simulink model "Central_locking"  (R2017b)
settings: Solver=VariableStepAuto  StartTime=0.0  StopTime=10.0  RelTol=1e-3
undefined symbols (not defined in the file): sigbuilder_block
settings Model: Creator=ECoDe_user18  LastModifiedBy=ECoDe_user11
settings ConfigComp: CovEnable=on  RecordCoverage=on  CovMetricSettings=dcmwe  CovModelRefEnable=on  CovExternalEMLEnable=off  CovSFcnEnable=off

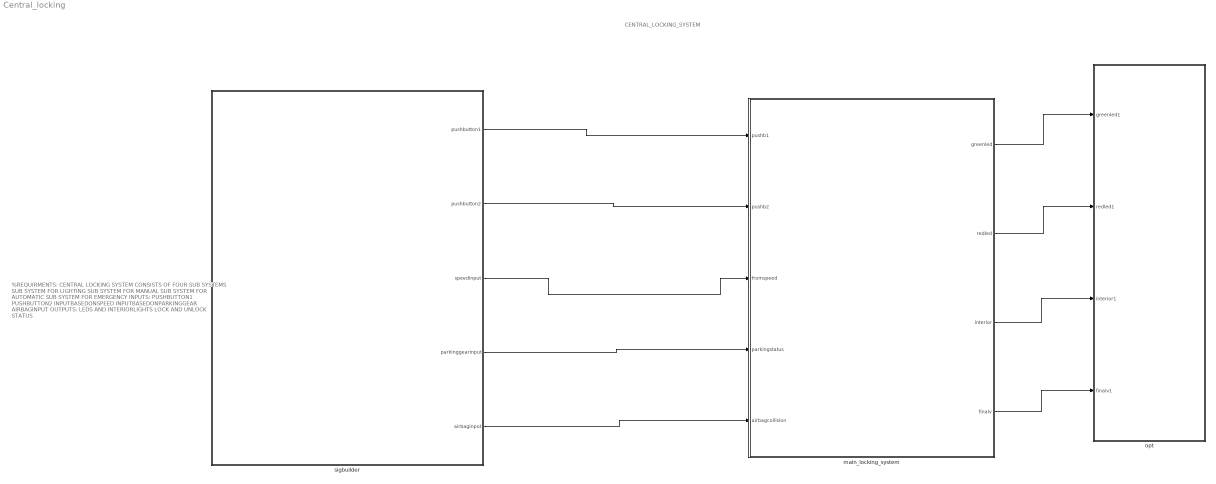
== system Central_locking ==
  note: %REQUIRMENTS:
      | CENTRAL LOCKING SYSTEM
      | CONSISTS OF FOUR SUB SYSTEMS
      | SUB SYSTEM FOR LIGHTING
      | SUB SYSTEM FOR MANUAL
      | SUB SYSTEM FOR AUTOMATIC
      | SUB SYSTEM FOR EMERGENCY
      | INPUTS:
      | PUSHBUTTON1
      | PUSHBUTTON2
      | INPUTBASEDONSPEED
      | INPUTBASEDONPARKINGGEAR
      | AIRBAGINPUT
      | OUTPUTS:
      | LEDS AND INTERIORLIGHTS
      | LOCK AND UNLOCK STATUS
  note: CENTRAL_LOCKING_SYSTEM
  main_locking_system : Subsystem
  opt : Subsystem
  sigbuilder : Subsystem
  wires:
  sigbuilder/1(pushbutton1) -> main_locking_system/1(pushb1)
  sigbuilder/2(pushbutton2) -> main_locking_system/2(pushb2)
  sigbuilder/3(speedinput) -> main_locking_system/3(fromspeed)
  sigbuilder/4(parkinggearinput) -> main_locking_system/4(parkingstatus)
  sigbuilder/5(airbaginput) -> main_locking_system/5(airbagcollision)
  main_locking_system/1(greenled) -> opt/1(greenled1)
  main_locking_system/2(redled) -> opt/2(redled1)
  main_locking_system/3(interior) -> opt/3(interior1)
  main_locking_system/4(finalv) -> opt/4(finalv1)

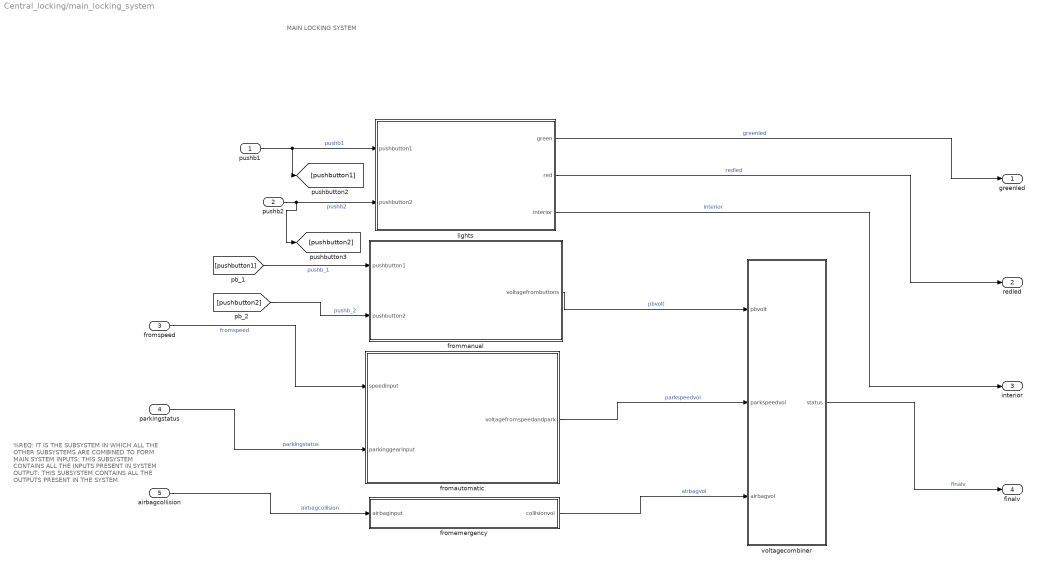
== system Central_locking/main_locking_system ==
  note: %REQ:
      | IT IS THE SUBSYSTEM IN
      | WHICH ALL THE OTHER SUBSYSTEMS
      | ARE COMBINED TO FORM MAIN SYSTEM
      | INPUTS:
      | THIS SUBSYSTEM CONTAINS ALL THE
      | INPUTS PRESENT IN SYSTEM
      | OUTPUT:
      | THIS SUBSYSTEM CONTAINS ALL THE
      | OUTPUTS PRESENT IN  THE SYSTEM.
  note: MAIN LOCKING SYSTEM
  pushb1 : Inport
  pushb2 : Inport  Port=2
  fromspeed : Inport  Port=3
  parkingstatus : Inport  Port=4
  airbagcollision : Inport  Port=5
  fromautomatic : Subsystem
  fromemergency : Subsystem
  frommanual : Subsystem
  lights : Subsystem
  voltagecombiner : Subsystem
  greenled : Outport
  redled : Outport  Port=2
  interior : Outport  Port=3
  finalv : Outport  Port=4
  wires:
  pushb1/1 -> [pushbutton1], lights/1(pushbutton1)  "pushb1"
  voltagecombiner/1(status) -> finalv/1  "finalv"
  frommanual/1(voltagefrombuttons) -> voltagecombiner/1(pbvolt)  "pbvolt"
  airbagcollision/1 -> fromemergency/1(airbaginput)  "airbagcollision"
  fromautomatic/1(voltagefromspeedandpark) -> voltagecombiner/2(parkspeedvol)  "parkspeedvol"
  [pushbutton1] -> frommanual/1(pushbutton1)  "pushb_1"
  pushb2/1 -> [pushbutton2], lights/2(pushbutton2)  "pushb2"
  parkingstatus/1 -> fromautomatic/2(parkinggearinput)  "parkingstatus"
  fromspeed/1 -> fromautomatic/1(speedinput)  "fromspeed"
  lights/1(green) -> greenled/1  "greenled"
  lights/3(interior) -> interior/1  "interior"
  lights/2(red) -> redled/1  "redled"
  fromemergency/1(collisionvol) -> voltagecombiner/3(airbagvol)  "airbagvol"
  [pushbutton2] -> frommanual/2(pushbutton2)  "pushb_2"

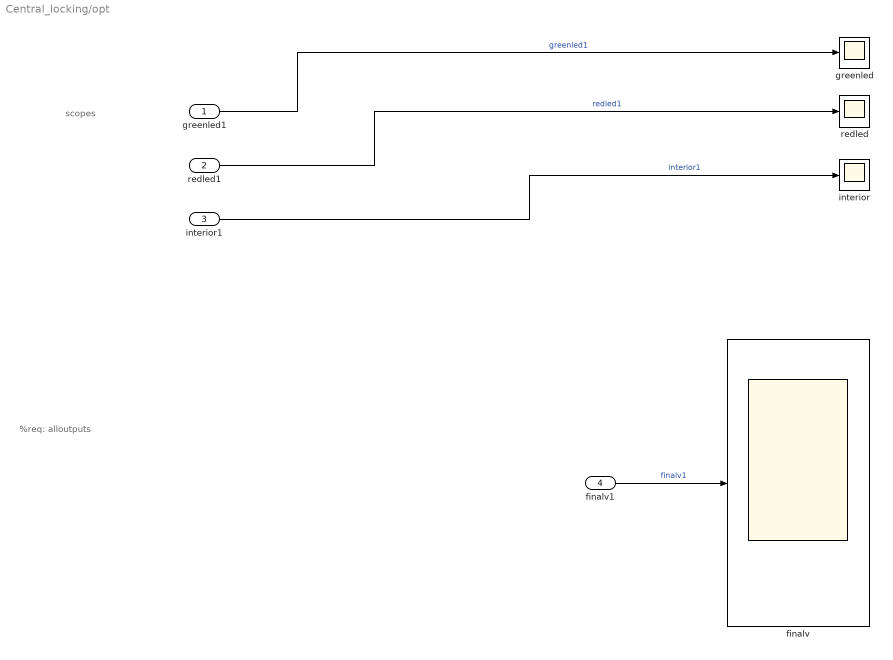
== system Central_locking/opt ==
  note: %req:
      | alloutputs
  note: scopes
  greenled1 : Inport
  redled1 : Inport  Port=2
  interior1 : Inport  Port=3
  finalv1 : Inport  Port=4
  finalv : Scope
  greenled : Scope
  interior : Scope
  redled : Scope
  wires:
  redled1/1 -> redled/1  "redled1"
  interior1/1 -> interior/1  "interior1"
  greenled1/1 -> greenled/1  "greenled1"
  finalv1/1 -> finalv/1  "finalv1"

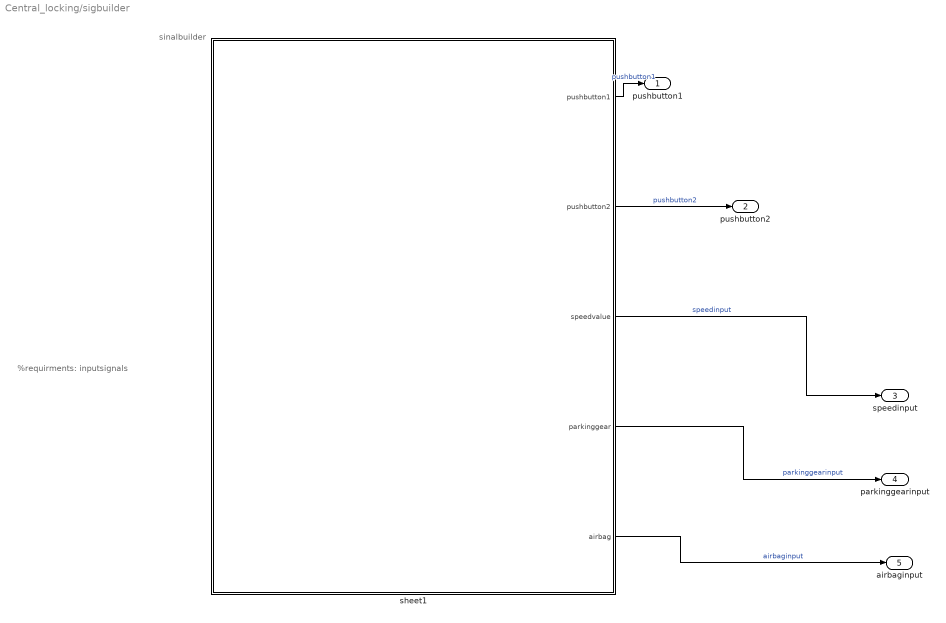
== system Central_locking/sigbuilder ==
  note: %requirments:
      | inputsignals
  note: sinalbuilder
  sheet1 : Subsystem  Tag=STV Subsys  LoadFcn=sigbuilder_block('load');  StartFcn=sigbuilder_block('start');  StopFcn=sigbuilder_block('stop');  ClipboardFcn=sigbuilder_block('clipboard');  mask(Sigbuilder block){tuvar=[0:10]}
      mask help: Simulink:masks:SigbuilderBlock_MD
      mask init:
      | if ~strcmp(get_param(bdroot(gcbh),'SimulationStatus'),'stopped') tuvar = sigbuilder_block('maskInit'); end
      settings: CopyFcn=sigbuilder_block('copy');  DeleteFcn=sigbuilder_block('delete');  ModelCloseFcn=sigbuilder_block('modelClose');  PreSaveFcn=sigbuilder_block('preSave');  PauseFcn=sigbuilder_block('pause');  ContinueFcn=sigbuilder_block('continue');  NameChangeFcn=sigbuilder_block('namechange');  OpenFcn=sigbuilder_block('open',[3 36 1018.5 456.75 ]);  CloseFcn=sigbuilder_block('close');
      mask Display: plot(0, 0, 100, 100,[2, 2, 32, 32, 2], [68, 8, 8, 68, 68],[32, 2], [38, 38], [32, 19, 2],[53, 60, 44], [32, 17, 17, 2],[16, 16, 31, 31]);txt = getActiveGroup(gcbh);text(2, 100, txt,'verticalAlignment', 'top');
  pushbutton1 : Outport
  pushbutton2 : Outport  Port=2
  speedinput : Outport  Port=3
  parkinggearinput : Outport  Port=4
  airbaginput : Outport  Port=5
  wires:
  sheet1/4(parkinggear) -> parkinggearinput/1  "parkinggearinput"
  sheet1/3(speedvalue) -> speedinput/1  "speedinput"
  sheet1/2(pushbutton2) -> pushbutton2/1  "pushbutton2"
  sheet1/5(airbag) -> airbaginput/1  "airbaginput"
  sheet1/1(pushbutton1) -> pushbutton1/1  "pushbutton1"

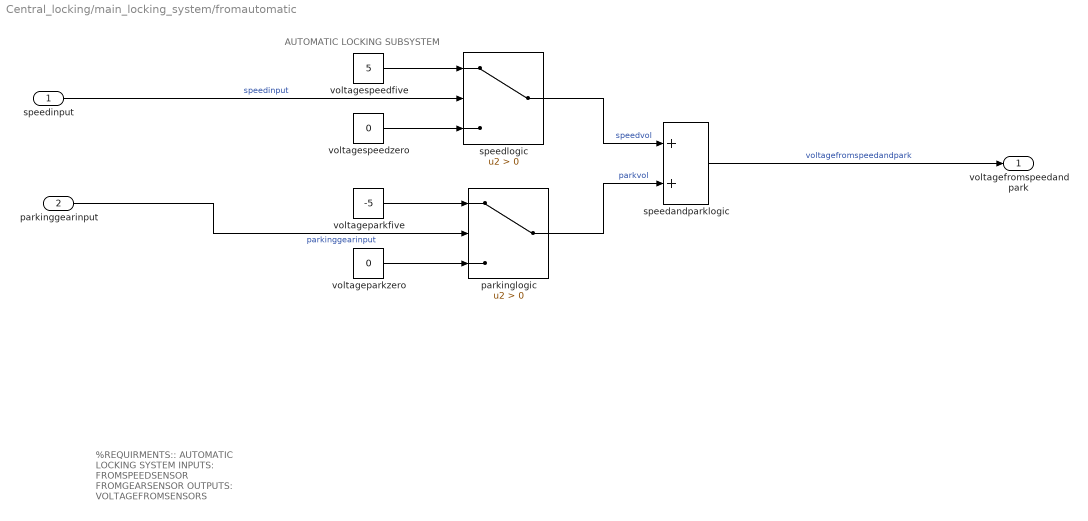
== system Central_locking/main_locking_system/fromautomatic ==
  note: AUTOMATIC LOCKING SUBSYSTEM
  note: %REQUIRMENTS::
      | AUTOMATIC LOCKING SYSTEM
      | INPUTS:
      | FROMSPEEDSENSOR
      | FROMGEARSENSOR
      | OUTPUTS:
      | VOLTAGEFROMSENSORS
  speedinput : Inport
  parkinggearinput : Inport  Port=2
  parkinglogic : Switch  Criteria=u2 > Threshold
  speedandparklogic : Sum
  speedlogic : Switch  Criteria=u2 > Threshold
  voltageparkfive : Constant  Value=-5
  voltageparkzero : Constant  Value=0
  voltagespeedfive : Constant  Value=5
  voltagespeedzero : Constant  Value=0
  voltagefromspeedandpark : Outport
  wires:
  speedinput/1 -> speedlogic/2  "speedinput"
  voltagespeedzero/1 -> speedlogic/3
  speedlogic/1 -> speedandparklogic/1  "speedvol"
  parkinglogic/1 -> speedandparklogic/2  "parkvol"
  parkinggearinput/1 -> parkinglogic/2  "parkinggearinput"
  voltageparkzero/1 -> parkinglogic/3
  voltageparkfive/1 -> parkinglogic/1
  voltagespeedfive/1 -> speedlogic/1
  speedandparklogic/1 -> voltagefromspeedandpark/1  "voltagefromspeedandpark"

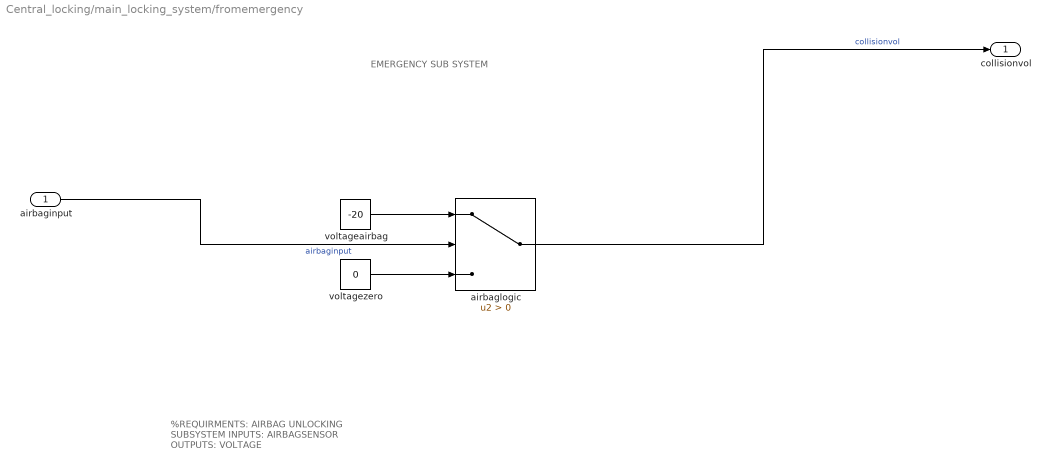
== system Central_locking/main_locking_system/fromemergency ==
  note: EMERGENCY SUB SYSTEM
  note: %REQUIRMENTS:
      | AIRBAG UNLOCKING SUBSYSTEM
      | INPUTS:
      | AIRBAGSENSOR
      | OUTPUTS:
      | VOLTAGE
  airbaginput : Inport
  airbaglogic : Switch  Criteria=u2 > Threshold
  voltageairbag : Constant  Value=-20
  voltagezero : Constant  Value=0
  collisionvol : Outport
  wires:
  voltagezero/1 -> airbaglogic/3
  airbaglogic/1 -> collisionvol/1  "collisionvol"
  voltageairbag/1 -> airbaglogic/1
  airbaginput/1 -> airbaglogic/2  "airbaginput"

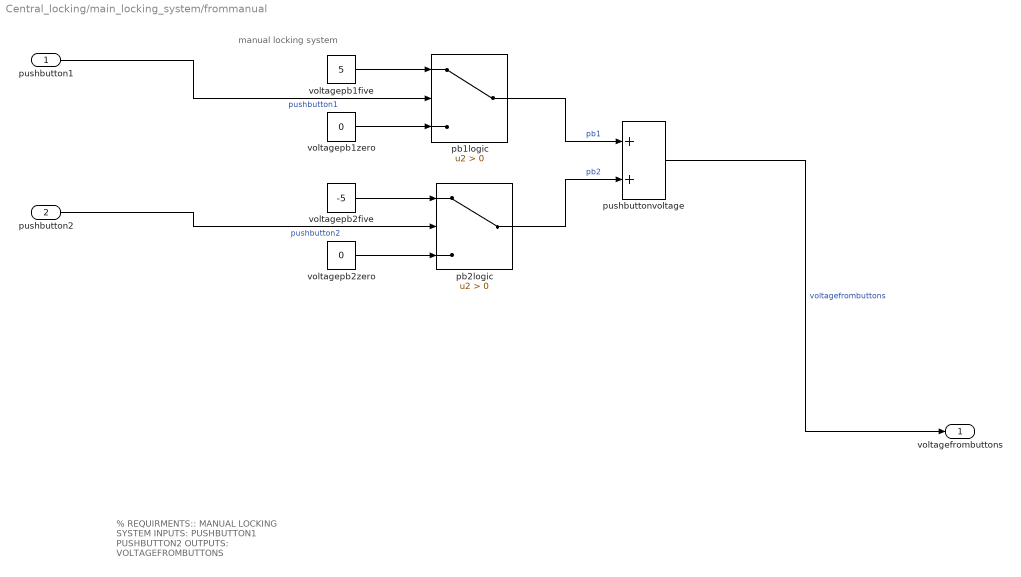
== system Central_locking/main_locking_system/frommanual ==
  note: manual locking system
  note: % REQUIRMENTS::
      | MANUAL LOCKING SYSTEM
      | INPUTS:
      | PUSHBUTTON1
      | PUSHBUTTON2
      | OUTPUTS:
      | VOLTAGEFROMBUTTONS
  pushbutton1 : Inport
  pushbutton2 : Inport  Port=2
  pb1logic : Switch  Criteria=u2 > Threshold
  pb2logic : Switch  Criteria=u2 > Threshold
  pushbuttonvoltage : Sum
  voltagepb1five : Constant  Value=5
  voltagepb1zero : Constant  Value=0
  voltagepb2five : Constant  Value=-5
  voltagepb2zero : Constant  Value=0
  voltagefrombuttons : Outport
  wires:
  pushbutton2/1 -> pb2logic/2  "pushbutton2"
  voltagepb1five/1 -> pb1logic/1
  pushbutton1/1 -> pb1logic/2  "pushbutton1"
  voltagepb1zero/1 -> pb1logic/3
  pb2logic/1 -> pushbuttonvoltage/2  "pb2"
  voltagepb2five/1 -> pb2logic/1
  voltagepb2zero/1 -> pb2logic/3
  pb1logic/1 -> pushbuttonvoltage/1  "pb1"
  pushbuttonvoltage/1 -> voltagefrombuttons/1  "voltagefrombuttons"

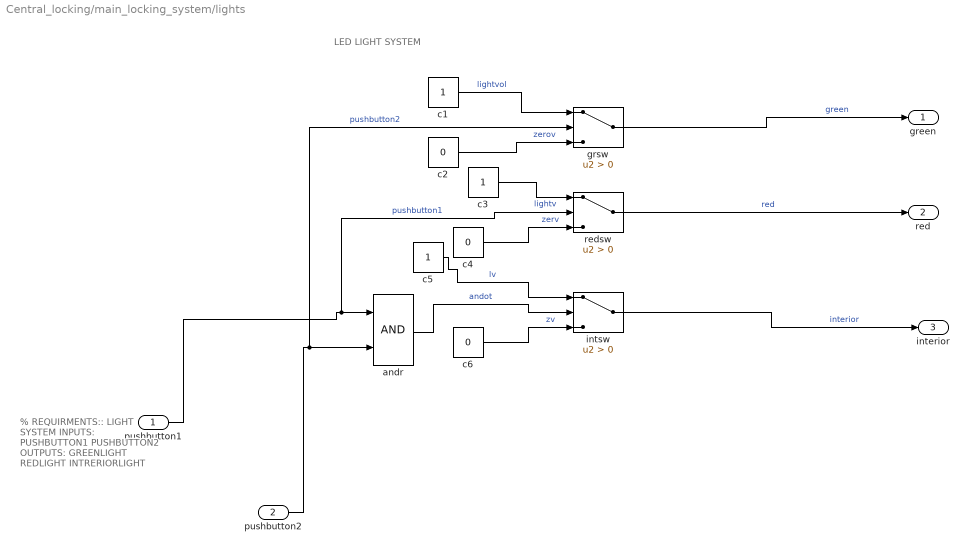
== system Central_locking/main_locking_system/lights ==
  note: LED LIGHT SYSTEM
  note: % REQUIRMENTS::
      | LIGHT SYSTEM
      | INPUTS:
      | PUSHBUTTON1
      | PUSHBUTTON2
      | OUTPUTS:
      | GREENLIGHT
      | REDLIGHT
      | INTRERIORLIGHT
  pushbutton1 : Inport
  pushbutton2 : Inport  Port=2
  andr : Logic  AllPortsSameDT=off  OutDataTypeStr=boolean
  c1 : Constant
  c2 : Constant  Value=0
  c3 : Constant
  c4 : Constant  Value=0
  c5 : Constant
  c6 : Constant  Value=0
  grsw : Switch  Criteria=u2 > Threshold
  intsw : Switch  Criteria=u2 > Threshold
  redsw : Switch  Criteria=u2 > Threshold
  green : Outport
  red : Outport  Port=2
  interior : Outport  Port=3
  wires:
  c6/1 -> intsw/3  "zv"
  c5/1 -> intsw/1  "lv"
  andr/1 -> intsw/2  "andot"
  pushbutton1/1 -> redsw/2, andr/1  "pushbutton1"
  intsw/1 -> interior/1  "interior"
  pushbutton2/1 -> grsw/2, andr/2  "pushbutton2"
  grsw/1 -> green/1  "green"
  c1/1 -> grsw/1  "lightvol"
  redsw/1 -> red/1  "red"
  c2/1 -> grsw/3  "zerov"
  c3/1 -> redsw/1  "lightv"
  c4/1 -> redsw/3  "zerv"

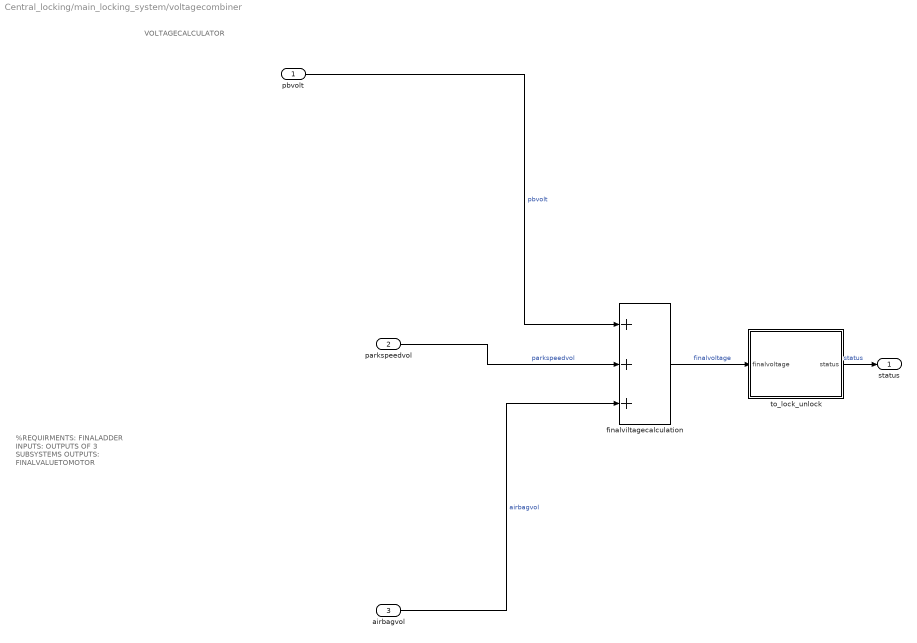
== system Central_locking/main_locking_system/voltagecombiner ==
  note: VOLTAGECALCULATOR
  note: %REQUIRMENTS:
      | FINALADDER
      | INPUTS:
      | OUTPUTS OF 3 SUBSYSTEMS
      | OUTPUTS:
      | FINALVALUETOMOTOR
  pbvolt : Inport
  parkspeedvol : Inport  Port=2
  airbagvol : Inport  Port=3
  finalviltagecalculation : Sum  Inputs=+++
  to_lock_unlock : Stateflow chart  TreatAsAtomicUnit=on
  status : Outport
  wires:
  parkspeedvol/1 -> finalviltagecalculation/2  "parkspeedvol"
  airbagvol/1 -> finalviltagecalculation/3  "airbagvol"
  pbvolt/1 -> finalviltagecalculation/1  "pbvolt"
  to_lock_unlock/1(status) -> status/1  "status"
  finalviltagecalculation/1 -> to_lock_unlock/1(finalvoltage)  "finalvoltage"

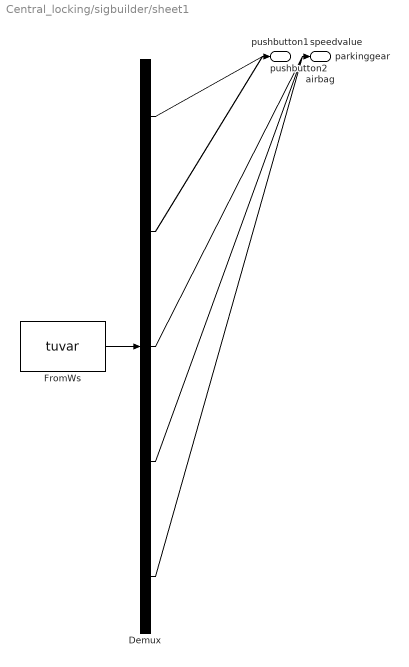
== system Central_locking/sigbuilder/sheet1 ==
  Demux : Demux  Tag=STV Demux  Outputs=5
  FromWs : FromWorkspace  Tag=STV FromWs  VariableName=tuvar  SampleTime=0
      SigBuilderData=|
      | common.afterFinalStr = 'Extrapolate'
      | common.sampleTime = 0
      | dataSet.timeRange = [0 9]
      | dataSet.name = 'Sheet1'
      | sbobj.Name = 'Signal Builder'
      | sbobj.Groups.Name = 'Sheet1'
      | sbobj.Groups.Signals(1).Name = 'pushbutton1'
      | sbobj.Groups.Signals(1).XData = [0 1 1 2 2 3 3 4 5 6 7 8 8 9]
      | sbobj.Groups.Signals(1).YData = [1 1 0 0 1 1 0 0 0 0 0 0 1 1]
      | sbobj.Groups.Signals(2).Name = 'pushbutton2'
      | sbobj.Groups.Signals(2).XData = [0 1 1 2 3 3 4 5 6 7 8 9]
      | sbobj.Groups.Signals(2).YData = [0 0 1 1 1 0 0 0 0 0 0 0]
      | sbobj.Groups.Signals(3).Name = 'speedvalue'
      | sbobj.Groups.Signals(3).XData = [0 1 2 3 3 4 4 5 5 6 7 7 8 8 9]
      | sbobj.Groups.Signals(3).YData = [0 0 0 0 1 1 0 0 1 1 1 0 0 1 1]
      | sbobj.Groups.Signals(4).Name = 'parkinggear'
      | sbobj.Groups.Signals(4).XData = [0 1 2 3 4 4 5 6 7 7 8 9]
      | sbobj.Groups.Signals(4).YData = [0 0 0 0 0 1 1 1 1 0 0 0]
      | sbobj.Groups.Signals(5).Name = 'airbag'
      | sbobj.Groups.Signals(5).XData = [0 1 2 3 4 5 6 6 7 8 9]
      | sbobj.Groups.Signals(5).YData = [0 0 0 0 0 0 0 1 1 1 1]
      | sbobj.Groups.TimeRange = [0 9]
  pushbutton1 : Outport  Tag=STV Outport
  pushbutton2 : Outport  Tag=STV Outport  Port=2
  speedvalue : Outport  Tag=STV Outport  Port=3
  parkinggear : Outport  Tag=STV Outport  Port=4
  airbag : Outport  Tag=STV Outport  Port=5
  wires:
  FromWs/1 -> Demux/1
  Demux/1 -> pushbutton1/1
  Demux/2 -> pushbutton2/1
  Demux/3 -> speedvalue/1
  Demux/4 -> parkinggear/1
  Demux/5 -> airbag/1

== stateflow chart Central_locking/main_locking_system/voltagecombiner/to_lock_unlock ==
  note: LOGICTOLOCKANDUNLOCK
  note: %REQ:
      | here depending on the
      | value of finalvalue from adder
      | we get the status from this
      | chart depending on conditions
      | given.
      | input is 0 then status is 0
      | input is +ve then status 1
      | input is -ve then status -1
  (default) -> (junction 1)
  (junction 1) -> (junction 5) [order 2] : [finalvoltage>0]{status=1}
  (junction 1) -> (junction 8) [order 3] : [finalvoltage<0]{status=-1}
  (junction 1) -> (junction 3) [order 1] : [finalvoltage==0]{status=0}
  (junction 5) -> (junction 13)
  (junction 8) -> (junction 13)
  (junction 3) -> (junction 13)
  data: finalvoltage input; status output
